simulink model "LGPR_exp"  (R2022a)
settings: Solver=ode1  StartTime=0.0  StopTime=20  FixedStep=0.001  RelTol=1e-3
libraries: roblocks x1
settings Model: Creator=DELL  LastModifiedBy=qinyi
settings DebuggingCC: UnconnectedInputMsg=warning  UnconnectedOutputMsg=warning  UnconnectedLineMsg=warning
settings RTWCC: DLArmComputeVersion=19.05

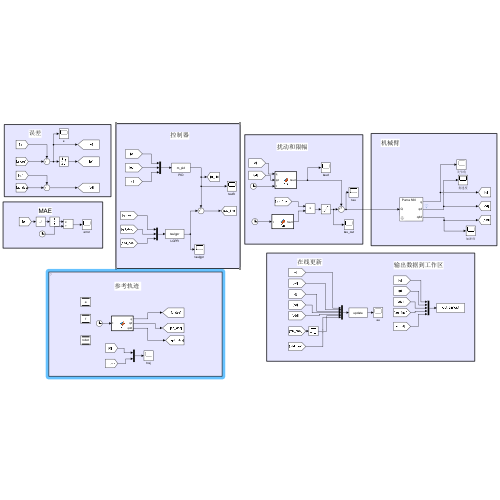
[thumbnail: Simulink's stored preview of the top-level diagram]
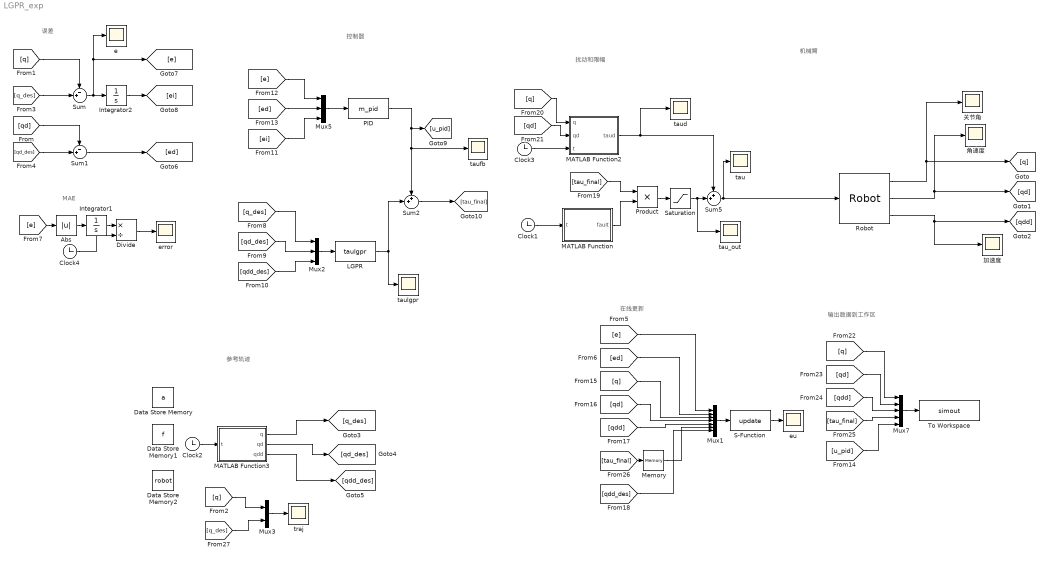
== system LGPR_exp ==
  note: 在线更新
  note: MAE
  note: 机械臂
  note: 扰动和限幅
  note: 控制器
  note: 误差
  note: 参考轨迹
  note: 输出数据到工作区
  Abs : Abs  SaturateOnIntegerOverflow=off
  Clock{1..4} (4 alike) : Clock
  Data Store Memory : DataStoreMemory  DataStoreName=a  ReadBeforeWriteMsg=warning  WriteAfterWriteMsg=warning  WriteAfterReadMsg=warning  InitialValue=rand(10,6)  ShowAdditionalParam=off  OutDataTypeStr=double
  Data Store Memory1 : DataStoreMemory  DataStoreName=f  ReadBeforeWriteMsg=warning  WriteAfterWriteMsg=warning  WriteAfterReadMsg=warning  InitialValue=rand(10,6)  ShowAdditionalParam=off  OutDataTypeStr=double
  Data Store Memory2 : DataStoreMemory  DataStoreName=robot  ReadBeforeWriteMsg=warning  WriteAfterWriteMsg=warning  WriteAfterReadMsg=warning  InitialValue=rand(10,6)  ShowAdditionalParam=off  OutDataTypeStr=double
  Divide : Product  Inputs=*/
  Integrator1 : Integrator
  Integrator2 : Integrator  LimitOutput=on  UpperSaturationLimit=0.01  LowerSaturationLimit=-0.01
  LGPR : S-Function  FunctionName=taulgpr  Parameters=p560  SFunctionDeploymentMode=off  EnableBusSupport=off
  MATLAB Function : MATLAB Function  TreatAsAtomicUnit=on
  MATLAB Function2 : MATLAB Function  TreatAsAtomicUnit=on
  MATLAB Function3 : MATLAB Function  TreatAsAtomicUnit=on
  Memory : Memory
  Mux1 : Mux  Inputs=7
  Mux2 : Mux  Inputs=3
  Mux3 : Mux  Inputs=2
  Mux5 : Mux  Inputs=3
  Mux7 : Mux  Inputs=5
  PID : S-Function  FunctionName=m_pid  SFunctionDeploymentMode=off  EnableBusSupport=off
  Product : Product
  Robot : roblocks/Arm/Robot  robot=p560  q0=[90 0 30 60 30 30]*pi/180
      link override Integrator: InitialCondition=0
      link override Integrator1: InitialCondition=[0 90 -90 30 0 0]'*pi/180
      link override S-Function: Parameters=p560
  S-Function : S-Function  FunctionName=update  SFunctionDeploymentMode=off  EnableBusSupport=off
  Saturation : Saturate  UpperLimit=400  LowerLimit=-400
  Sum : Sum  Inputs=-+|
  Sum1 : Sum  Inputs=-+|
  Sum2 : Sum  Inputs=++|
  Sum5 : Sum  Inputs=++|
  To Workspace : ToWorkspace  VariableName=simout  SaveFormat=Timeseries  SampleTime=-1
  e : Scope
  error : Scope
  eu : Scope
  tau : Scope
  tau_out : Scope
  taud : Scope
  taufb : Scope
  taulgpr : Scope
  traj : Scope
  关节角 : Scope
  加速度 : Scope
  角速度 : Scope
  wires:
  Sum/1 -> Integrator2/1, e/1, [e]
  Sum1/1 -> [ed]
  Clock1/1 -> MATLAB Function/1(t)
  Clock3/1 -> MATLAB Function2/3(t)
  Mux2/1 -> LGPR/1
  Sum5/1 -> Robot/1, tau/1
  Abs/1 -> Integrator1/1
  Integrator1/1 -> Divide/1
  Divide/1 -> error/1
  Mux5/1 -> PID/1
  S-Function/1 -> eu/1
  Mux7/1 -> To Workspace/1
  LGPR/1 -> Sum2/2, taulgpr/1
  Memory/1 -> Mux1/6
  Mux1/1 -> S-Function/1
  Robot/1 -> [q], 关节角/1
  Robot/2 -> [qd], 角速度/1
  Robot/3 -> [qdd], 加速度/1
  Integrator2/1 -> [ei]
  MATLAB Function/1(fault) -> Product/2
  Clock2/1 -> MATLAB Function3/1(t)
  MATLAB Function3/1(q) -> [q_des]
  MATLAB Function3/2(qd) -> [qd_des]
  MATLAB Function3/3(qdd) -> [qdd_des]
  Clock4/1 -> Divide/2
  [q] -> Sum/1
  [qd] -> Sum1/1
  [q_des] -> Sum/2
  [qd_des] -> Sum1/2
  [e] -> Mux1/1
  [ed] -> Mux1/2
  [e] -> Abs/1
  [q_des] -> Mux2/1
  [qd_des] -> Mux2/2
  [qdd_des] -> Mux2/3
  [e] -> Mux5/1
  [ed] -> Mux5/2
  [ei] -> Mux5/3
  PID/1 -> taufb/1, Sum2/1, [u_pid]
  [u_pid] -> Mux7/5
  [q] -> Mux1/3
  [qd] -> Mux1/4
  [qdd] -> Mux1/5
  [qdd_des] -> Mux1/7
  Sum2/1 -> [tau_final]
  [tau_final] -> Product/1
  [q] -> MATLAB Function2/1(q)
  [qd] -> MATLAB Function2/2(qd)
  MATLAB Function2/1(taud) -> taud/1, Sum5/1
  [q] -> Mux7/1
  [qd] -> Mux7/2
  [qdd] -> Mux7/3
  [tau_final] -> Mux7/4
  [tau_final] -> Memory/1
  Product/1 -> Saturation/1
  Saturation/1 -> tau_out/1, Sum5/2
  Mux3/1 -> traj/1
  [q] -> Mux3/1
  [q_des] -> Mux3/2

== matlab function LGPR_exp/MATLAB Function2 ==
  settings: updateMethod=DISCRETE
  data: q input; qd input; t input; taud output; a data_store_memory; f data_store_memory
function taud  = dis(q,qd,t)
rng(1);

taud=[30; 30 ;30 ;10 ;10 ;10]*sin(0.3*pi*t)+[5; 5 ;5 ;5 ;5 ;5].*sin(q).*qd+[1; 1; 1; 1; 1; 1].*qd+randn(6,1);

%taud = [30; 30 ;30 ;10 ;10 ;10]*sin(0.3*pi*t)+[10; 10 ;10 ;5 ;5 ;5].*sin(q).*qd+[2; 2 ;2 ;1; 1 ;1].*qd+randn(6,1);

if(t<10)
    taud=0*taud;
else
    taud=1*taud;
end

== matlab function LGPR_exp/MATLAB Function ==
  data: t input; fault output
 function fault = fcn(t)
if(t>10)
    fault = 0.5+0.5*exp(-0.3*(t-10));
else
    fault=1;
end

== matlab function LGPR_exp/MATLAB Function3 ==
  settings: updateMethod=DISCRETE
  data: t input; q output; qd output; qdd output; a data_store_memory; f data_store_memory
function [q,qd,qdd] = fcn(t)

fq=1*ones(1,6);
B=[80 70 70 70 50 120]*pi/180;
q=[B.*sin(fq*t)]'+[0 90 -90 30 0 0]'*pi/180;
qd=[B.*fq.*cos(fq*t)]';
qdd=[-B.*fq.*fq.*sin(fq*t)]';
